simulink model "simulatedData"  (R2013a)
settings: Solver=ode45  StartTime=0.0  StopTime=10.0  MaxStep=0.01  RelTol=1e-3
values from neighbouring files (symbols this model uses):
  gpsSampleTime = 0.1    [runPositionFilter.m]    (also in workspace.mat)
  sampleTime = 0.01    [runPositionFilter.m]    (also in runtracklsq.m = mydata.sampleTime; workspace.mat)
libraries: simulink x3
settings Model: Creator=User  LastModifiedBy=User

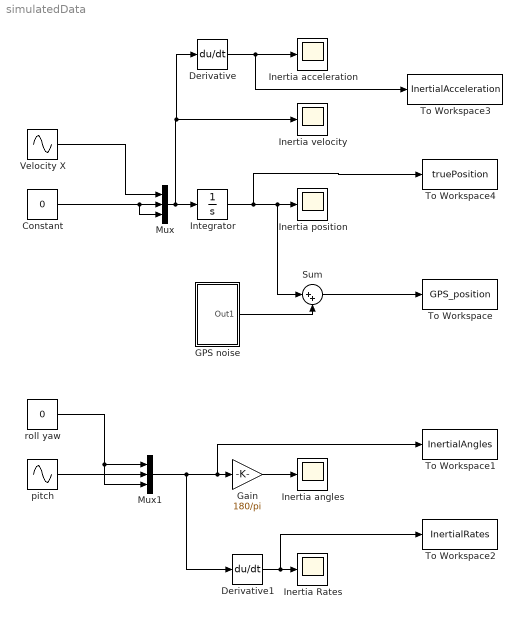
== system simulatedData ==
  Constant : Constant  Value=0
  Derivative : Derivative
  Derivative1 : Derivative
  "GPS noise " : Subsystem
  Gain : Gain  Gain=180/pi
  "Inertia Rates " : Scope
      settings: SaveName=ScopeData4
  Inertia acceleration : Scope
      settings: SaveName=ScopeData3
  Inertia angles : Scope
      settings: SaveName=ScopeData2
  Inertia position : Scope
  Inertia velocity : Scope
  Integrator : Integrator
  Mux : Mux  Inputs=3
  Mux1 : Mux  Inputs=3
  Sum : Sum  Inputs=|++
  To Workspace : ToWorkspace  VariableName=GPS_position  SampleTime=gpsSampleTime  SaveFormat=Structure With Time
  To Workspace1 : ToWorkspace  VariableName=InertialAngles  SampleTime=sampleTime  SaveFormat=Structure With Time
  To Workspace2 : ToWorkspace  VariableName=InertialRates  SampleTime=sampleTime  SaveFormat=Structure With Time
  To Workspace3 : ToWorkspace  VariableName=InertialAcceleration  SampleTime=sampleTime  SaveFormat=Structure With Time
  To Workspace4 : ToWorkspace  VariableName=truePosition  SampleTime=sampleTime  SaveFormat=Structure With Time
  Velocity X : Sin  Amplitude=8  Bias=20  SampleTime=0
  pitch : Sin  Amplitude=0.25  Frequency=10
  roll yaw : Constant  Value=0
  wires:
  Velocity X/1 -> Mux/1
  Mux/1 -> Derivative/1, Inertia velocity/1, Integrator/1
  Integrator/1 -> To Workspace4/1, Sum/1, Inertia position/1
  Constant/1 -> Mux/3, Mux/2
  Sum/1 -> To Workspace/1
  "GPS noise "/1(Out1) -> Sum/2
  pitch/1 -> Mux1/2
  roll yaw/1 -> Mux1/3, Mux1/1
  Mux1/1 -> Derivative1/1, To Workspace1/1, Gain/1
  Gain/1 -> Inertia angles/1
  Derivative/1 -> To Workspace3/1, Inertia acceleration/1
  Derivative1/1 -> To Workspace2/1, "Inertia Rates "/1

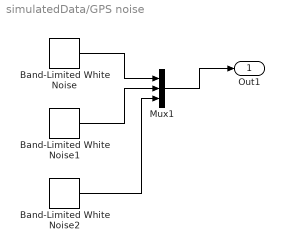
== system simulatedData/GPS noise  ==
  Band-Limited White Noise : simulink/Sources/Band-Limited White Noise  Cov=[0.001]*gpsSampleTime*1  Ts=gpsSampleTime  seed=[23341]
  Band-Limited White Noise1 : simulink/Sources/Band-Limited White Noise  Cov=[0.001]*gpsSampleTime*1  Ts=gpsSampleTime  seed=[23341]
  Band-Limited White Noise2 : simulink/Sources/Band-Limited White Noise  Cov=[0.001]*gpsSampleTime*1  Ts=gpsSampleTime  seed=[23341]
  Mux1 : Mux  Inputs=3
  Out1 : Outport
  wires:
  Mux1/1 -> Out1/1
  Band-Limited White Noise1/1 -> Mux1/2
  Band-Limited White Noise2/1 -> Mux1/3
  Band-Limited White Noise/1 -> Mux1/1
